simulink library "wheelSpeed_lib"  (R2023b)
settings: Solver=VariableStepAuto  StartTime=0.0  StopTime=10.0  RelTol=1e-3
undefined symbols (not defined in the file): raptor_xcp_function
libraries: Raptor_lib x50, simulink x6, $bdroot x4
settings Model: Creator=serga  LastModifiedBy=serga
settings OptimizationCC: ReuseModelBlockBuffer=off

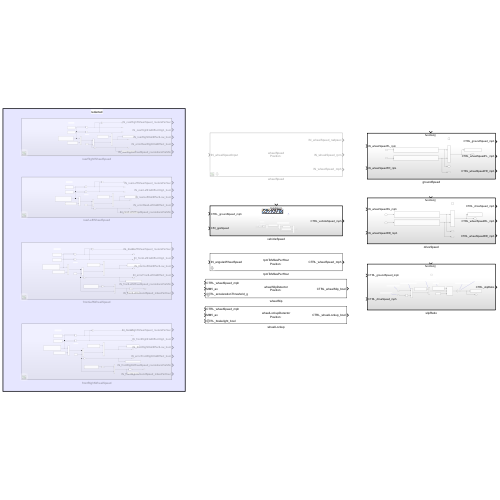
[thumbnail: Simulink's stored preview of the top-level diagram]
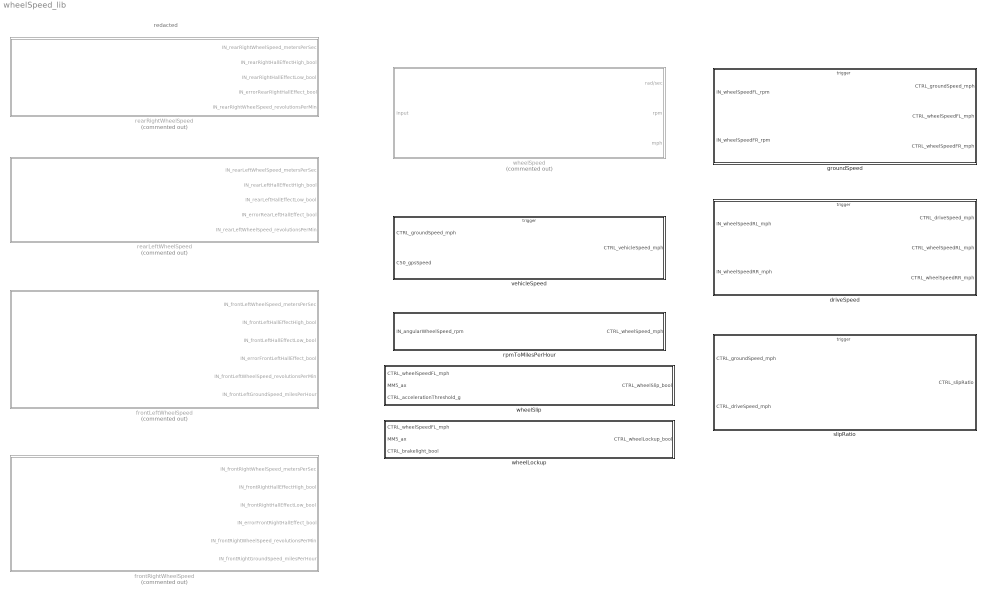
== system wheelSpeed_lib ==
  note: redacted
  driveSpeed : Subsystem  TreatAsAtomicUnit=on
  frontLeftWheelSpeed : Subsystem  Commented=on
  frontRightWheelSpeed : Subsystem  Commented=on
  groundSpeed : Subsystem  TreatAsAtomicUnit=on
  rearLeftWheelSpeed : Subsystem  Commented=on
  rearRightWheelSpeed : Subsystem  Commented=on
  rpmToMilesPerHour : Subsystem  mask{pos=''}
      mask prompts: pos "Position"
      mask Display:
      | disp(['rpmToMilesPerHour\n' ...
      |     'Position: ' pos]);
      | port_label('input', 1, ['IN_angularWheelSpeed' pos]);
      | port_label('output', 1, ['CTRL_wheelSpeed' pos '_mph']);
  slipRatio : Subsystem  TreatAsAtomicUnit=on
  vehicleSpeed : Subsystem
  wheelLockup : Subsystem  mask{pos=''}
      mask prompts: pos "Position"
      mask Display:
      | disp(['wheelLockupDetector\n' ...
      |     'Position: ' pos]);
      | port_label('input', 1, ['CTRL_wheelSpeed' pos '_mph']);
      | port_label('input', 2, 'MM5_ax');
      | port_label('input', 3, 'CTRL_brakelight_bool');
      | port_label('output', 1, ['CTRL_wheelLockup' pos '_bool']);
  wheelSlip : Subsystem  mask{pos=''}
      mask prompts: pos "Position"
      mask Display:
      | disp(['wheelSlipDetector\n' ...
      |     'Position: ' pos]);
      | port_label('input', 1, ['CTRL_wheelSpeed' pos '_mph']);
      | port_label('input', 2, 'MM5_ax');
      | port_label('input', 3, 'CTRL_accelerationThreshold_g');
      | port_label('output', 1, ['CTRL_wheelSlip' pos '_bool']);
  wheelSpeed : Subsystem  Commented=on  mask{pos=''}
      mask prompts: pos "Position"
      mask Display:
      | disp(['wheelSpeed\n' ...
      |     'Position: ' pos]);
      | port_label('input', 1, ['IN_wheelSpeedInput' pos]);
      | port_label('output', 1, ['IN_wheelSpeed' pos '_radpsec']);
      | port_label('output', 2, ['IN_wheelSpeed' pos '_rpm']);
      | port_label('output', 3, ['IN_wheelSpeed' pos '_mph']);

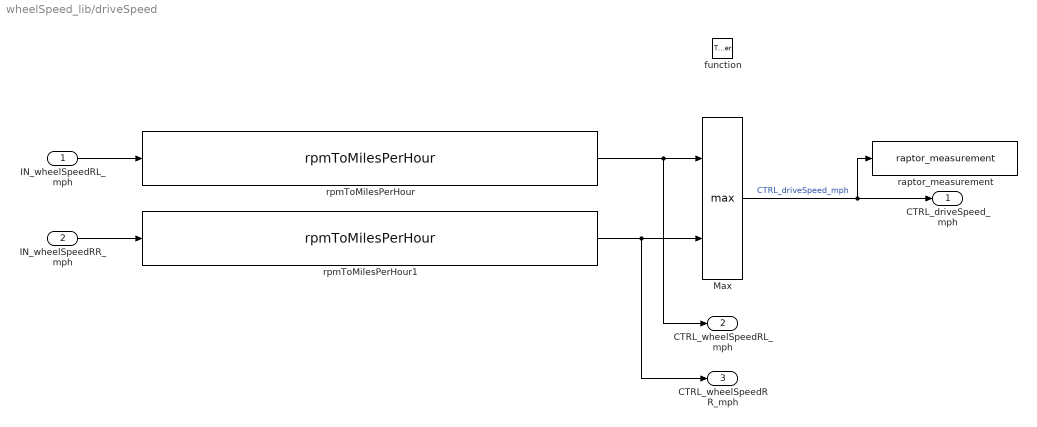
== system wheelSpeed_lib/driveSpeed ==
  IN_wheelSpeedRL_mph : Inport
  IN_wheelSpeedRR_mph : Inport  Port=2
  function : TriggerPort  TriggerType=function-call  VariantControl=(inherit)
  Max : MinMax  Function=max  Inputs=2
  raptor_measurement : Raptor_lib/Data Storage/raptor_measurement  paramName='DataName'  nameSource=Input Wire  calDispType=Number  calEnum={'False', 'True'}  calGain=1.0  calOffset=0.0  calMax=inf  calMin=-inf  calFormat='-1'  calUnit=''  calHelp=''  calAccess=1  calFunction=raptor_xcp_function(gcb)  calVisible=on
      settings: SourceProductName=Raptor
  rpmToMilesPerHour : $bdroot/rpmToMilesPerHour  pos='RL'
  rpmToMilesPerHour1 : $bdroot/rpmToMilesPerHour  pos='RR'
  CTRL_driveSpeed_mph : Outport
  CTRL_wheelSpeedRL_mph : Outport  Port=2
  CTRL_wheelSpeedRR_mph : Outport  Port=3
  wires:
  Max/1 -> raptor_measurement/1, CTRL_driveSpeed_mph/1  "CTRL_driveSpeed_mph"
  rpmToMilesPerHour/1 -> CTRL_wheelSpeedRL_mph/1, Max/1
  IN_wheelSpeedRL_mph/1 -> rpmToMilesPerHour/1
  rpmToMilesPerHour1/1 -> CTRL_wheelSpeedRR_mph/1, Max/2
  IN_wheelSpeedRR_mph/1 -> rpmToMilesPerHour1/1

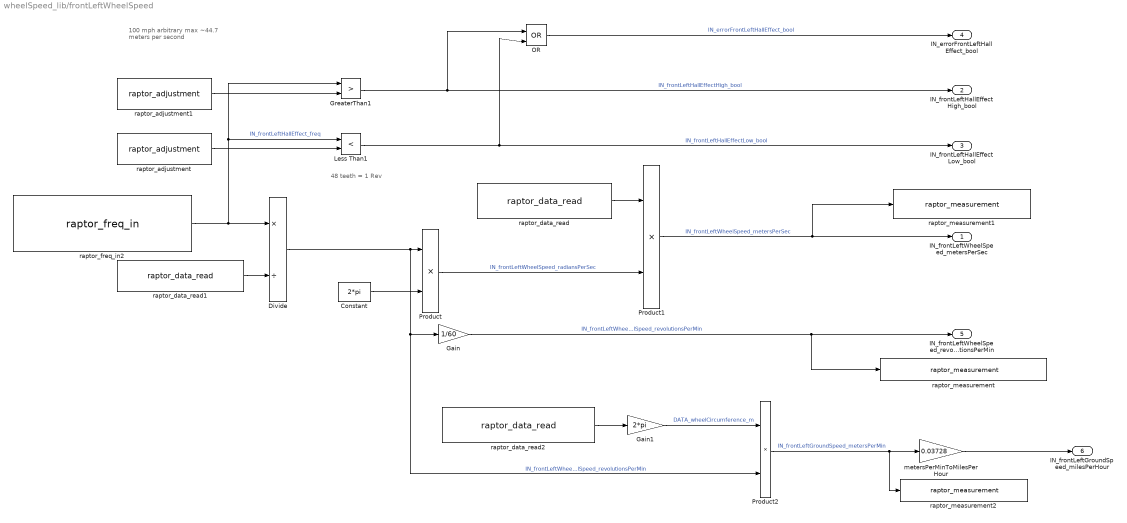
== system wheelSpeed_lib/frontLeftWheelSpeed ==
  note: 48 teeth = 1 Rev
  note: 100 mph arbitrary max
      | ~44.7 meters per second
  Constant : Constant  Value=2*pi
  Divide : Product  Inputs=*/
  Gain : Gain  Gain=1/60
  Gain1 : Gain  Gain=2*pi
  GreaterThan1 : RelationalOperator  Operator=>  OutDataTypeStr=boolean  RndMeth=Simplest  InputSameDT=off
  Less Than1 : RelationalOperator  Operator=<  OutDataTypeStr=boolean  RndMeth=Simplest  InputSameDT=off
  OR : Logic  Operator=OR  IconShape=distinctive  AllPortsSameDT=off  OutDataTypeStr=boolean
  Product : Product
  Product1 : Product
  Product2 : Product
  metersPerMinToMilesPerHour : Gain  Gain=0.03728
  raptor_adjustment : Raptor_lib/Data Storage/raptor_adjustment  paramName='IN_frontLeftHallEffectLow_freq'  nameSource=Parameter  initValue=0  dataType=single  storage=Calibration  calDispType=Number  calEnum={'False', 'True'}  calGain=1.0  calOffset=0.0  calMax=inf  calMin=-inf  calFormat='-1'  calUnit=''  calHelp=''  calAccess=1  calFunction=raptor_xcp_function(gcb)  calDispHeaders=off  calColHeaders={'Col1' 'Col2' 'Col3'}  calRowHeaders={'Row1' 'Row2' 'Row3'}
      settings: SourceProductName=Raptor
  raptor_adjustment1 : Raptor_lib/Data Storage/raptor_adjustment  paramName='IN_frontLeftHallEffectHigh_freq'  nameSource=Parameter  initValue=1680  dataType=single  storage=Calibration  calDispType=Number  calEnum={'False', 'True'}  calGain=1.0  calOffset=0.0  calMax=inf  calMin=-inf  calFormat='-1'  calUnit=''  calHelp=''  calAccess=1  calFunction=raptor_xcp_function(gcb)  calDispHeaders=off  calColHeaders={'Col1' 'Col2' 'Col3'}  calRowHeaders={'Row1' 'Row2' 'Row3'}
      settings: SourceProductName=Raptor
  raptor_data_read : Raptor_lib/Data Storage/raptor_data_read  dataName='DATA_unloadedWheelRadius_m'  dataShape=Scalar  idxSource=Input  idxRow=1  idxCol=1
      settings: SourceProductName=Raptor
  raptor_data_read1 : Raptor_lib/Data Storage/raptor_data_read  dataName='DATA_wheelTooth_ct'  dataShape=Scalar  idxSource=Input  idxRow=1  idxCol=1
      settings: SourceProductName=Raptor
  raptor_data_read2 : Raptor_lib/Data Storage/raptor_data_read  dataName='DATA_unloadedWheelRadius_m'  dataShape=Scalar  idxSource=Input  idxRow=1  idxCol=1
      settings: SourceProductName=Raptor
  raptor_freq_in2 : Raptor_lib/Input & Output/raptor_freq_in  minFreq='RAPTOR MASK DEFAULT'  resourceValues=INPUT41|INPUT42|INPUT43|INPUT44|INPUT45|(None)  resource=INPUT43  pullUDValues=[]  pullUD=[]  interfaceValues=[]  interface=[]  hasDuty=off  hasEdgeCount='RAPTOR MASK DEFAULT'
      settings: SourceProductName=Raptor
  raptor_measurement : Raptor_lib/Data Storage/raptor_measurement  paramName='DataName'  nameSource=Input Wire  calDispType=Number  calEnum={'False', 'True'}  calGain=1.0  calOffset=0.0  calMax=inf  calMin=-inf  calFormat='-1'  calUnit=''  calHelp=''  calAccess=1  calFunction=raptor_xcp_function(gcb)  calVisible=on
      settings: SourceProductName=Raptor
  raptor_measurement1 : Raptor_lib/Data Storage/raptor_measurement  paramName='DataName'  nameSource=Input Wire  calDispType=Number  calEnum={'False', 'True'}  calGain=1.0  calOffset=0.0  calMax=inf  calMin=-inf  calFormat='-1'  calUnit=''  calHelp=''  calAccess=1  calFunction=raptor_xcp_function(gcb)  calVisible=on
      settings: SourceProductName=Raptor
  raptor_measurement2 : Raptor_lib/Data Storage/raptor_measurement  paramName='DataName'  nameSource=Input Wire  calDispType=Number  calEnum={'False', 'True'}  calGain=1.0  calOffset=0.0  calMax=inf  calMin=-inf  calFormat='-1'  calUnit=''  calHelp=''  calAccess=1  calFunction=raptor_xcp_function(gcb)  calVisible=on
      settings: SourceProductName=Raptor
  IN_frontLeftWheelSpeed_metersPerSec : Outport
  IN_frontLeftHallEffectHigh_bool : Outport  Port=2
  IN_frontLeftHallEffectLow_bool : Outport  Port=3
  IN_errorFrontLeftHallEffect_bool : Outport  Port=4
  IN_frontLeftWheelSpeed_revolutionsPerMin : Outport  Port=5
  IN_frontLeftGroundSpeed_milesPerHour : Outport  Port=6
  wires:
  Product2/1 -> raptor_measurement2/1, metersPerMinToMilesPerHour/1  "IN_frontLeftGroundSpeed_metersPerMin"
  Divide/1 -> Product2/2, Gain/1, Product/1  "IN_frontLeftWheelSpeed_revolutionsPerMin"
  Gain1/1 -> Product2/1  "DATA_wheelCircumference_m"
  raptor_data_read/1 -> Product1/1
  raptor_data_read2/1 -> Gain1/1
  Less Than1/1 -> IN_frontLeftHallEffectLow_bool/1, OR/2  "IN_frontLeftHallEffectLow_bool"
  raptor_freq_in2/1 -> Less Than1/1, GreaterThan1/1, Divide/1  "IN_frontLeftHallEffect_freq"
  metersPerMinToMilesPerHour/1 -> IN_frontLeftGroundSpeed_milesPerHour/1
  Constant/1 -> Product/2
  raptor_adjustment/1 -> Less Than1/2
  OR/1 -> IN_errorFrontLeftHallEffect_bool/1  "IN_errorFrontLeftHallEffect_bool"
  raptor_adjustment1/1 -> GreaterThan1/2
  raptor_data_read1/1 -> Divide/2
  Product1/1 -> raptor_measurement1/1, IN_frontLeftWheelSpeed_metersPerSec/1  "IN_frontLeftWheelSpeed_metersPerSec"
  Gain/1 -> raptor_measurement/1, IN_frontLeftWheelSpeed_revolutionsPerMin/1  "IN_frontLeftWheelSpeed_revolutionsPerMin"
  Product/1 -> Product1/2  "IN_frontLeftWheelSpeed_radiansPerSec"
  GreaterThan1/1 -> IN_frontLeftHallEffectHigh_bool/1, OR/1  "IN_frontLeftHallEffectHigh_bool"

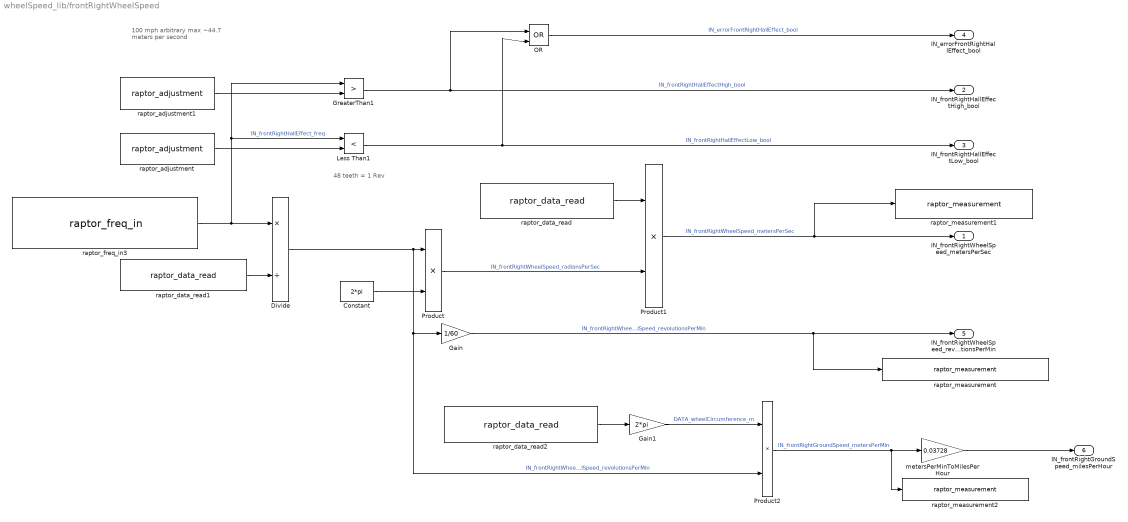
== system wheelSpeed_lib/frontRightWheelSpeed ==
  note: 100 mph arbitrary max
      | ~44.7 meters per second
  note: 48 teeth = 1 Rev
  Constant : Constant  Value=2*pi
  Divide : Product  Inputs=*/
  Gain : Gain  Gain=1/60
  Gain1 : Gain  Gain=2*pi
  GreaterThan1 : RelationalOperator  Operator=>  OutDataTypeStr=boolean  RndMeth=Simplest  InputSameDT=off
  Less Than1 : RelationalOperator  Operator=<  OutDataTypeStr=boolean  RndMeth=Simplest  InputSameDT=off
  OR : Logic  Operator=OR  IconShape=distinctive  AllPortsSameDT=off  OutDataTypeStr=boolean
  Product : Product
  Product1 : Product
  Product2 : Product
  metersPerMinToMilesPerHour : Gain  Gain=0.03728
  raptor_adjustment : Raptor_lib/Data Storage/raptor_adjustment  paramName='IN_frontRightHallEffectLow_freq'  nameSource=Parameter  initValue=0  dataType=single  storage=Calibration  calDispType=Number  calEnum={'False', 'True'}  calGain=1.0  calOffset=0.0  calMax=inf  calMin=-inf  calFormat='-1'  calUnit=''  calHelp=''  calAccess=1  calFunction=raptor_xcp_function(gcb)  calDispHeaders=off  calColHeaders={'Col1' 'Col2' 'Col3'}  calRowHeaders={'Row1' 'Row2' 'Row3'}
      settings: SourceProductName=Raptor
  raptor_adjustment1 : Raptor_lib/Data Storage/raptor_adjustment  paramName='IN_frontRightHallEffectHigh_freq'  nameSource=Parameter  initValue=1680  dataType=single  storage=Calibration  calDispType=Number  calEnum={'False', 'True'}  calGain=1.0  calOffset=0.0  calMax=inf  calMin=-inf  calFormat='-1'  calUnit=''  calHelp=''  calAccess=1  calFunction=raptor_xcp_function(gcb)  calDispHeaders=off  calColHeaders={'Col1' 'Col2' 'Col3'}  calRowHeaders={'Row1' 'Row2' 'Row3'}
      settings: SourceProductName=Raptor
  raptor_data_read : Raptor_lib/Data Storage/raptor_data_read  dataName='DATA_unloadedWheelRadius_m'  dataShape=Scalar  idxSource=Input  idxRow=1  idxCol=1
      settings: SourceProductName=Raptor
  raptor_data_read1 : Raptor_lib/Data Storage/raptor_data_read  dataName='DATA_wheelTooth_ct'  dataShape=Scalar  idxSource=Input  idxRow=1  idxCol=1
      settings: SourceProductName=Raptor
  raptor_data_read2 : Raptor_lib/Data Storage/raptor_data_read  dataName='DATA_unloadedWheelRadius_m'  dataShape=Scalar  idxSource=Input  idxRow=1  idxCol=1
      settings: SourceProductName=Raptor
  raptor_freq_in3 : Raptor_lib/Input & Output/raptor_freq_in  minFreq='RAPTOR MASK DEFAULT'  resourceValues=INPUT41|INPUT42|INPUT43|INPUT44|INPUT45|(None)  resource=INPUT44  pullUDValues=[]  pullUD=[]  interfaceValues=[]  interface=[]  hasDuty=off  hasEdgeCount='RAPTOR MASK DEFAULT'
      settings: SourceProductName=Raptor
  raptor_measurement : Raptor_lib/Data Storage/raptor_measurement  paramName='DataName'  nameSource=Input Wire  calDispType=Number  calEnum={'False', 'True'}  calGain=1.0  calOffset=0.0  calMax=inf  calMin=-inf  calFormat='-1'  calUnit=''  calHelp=''  calAccess=1  calFunction=raptor_xcp_function(gcb)  calVisible=on
      settings: SourceProductName=Raptor
  raptor_measurement1 : Raptor_lib/Data Storage/raptor_measurement  paramName='DataName'  nameSource=Input Wire  calDispType=Number  calEnum={'False', 'True'}  calGain=1.0  calOffset=0.0  calMax=inf  calMin=-inf  calFormat='-1'  calUnit=''  calHelp=''  calAccess=1  calFunction=raptor_xcp_function(gcb)  calVisible=on
      settings: SourceProductName=Raptor
  raptor_measurement2 : Raptor_lib/Data Storage/raptor_measurement  paramName='DataName'  nameSource=Input Wire  calDispType=Number  calEnum={'False', 'True'}  calGain=1.0  calOffset=0.0  calMax=inf  calMin=-inf  calFormat='-1'  calUnit=''  calHelp=''  calAccess=1  calFunction=raptor_xcp_function(gcb)  calVisible=on
      settings: SourceProductName=Raptor
  IN_frontRightWheelSpeed_metersPerSec : Outport
  IN_frontRightHallEffectHigh_bool : Outport  Port=2
  IN_frontRightHallEffectLow_bool : Outport  Port=3
  IN_errorFrontRightHallEffect_bool : Outport  Port=4
  IN_frontRightWheelSpeed_revolutionsPerMin : Outport  Port=5
  IN_frontRightGroundSpeed_milesPerHour : Outport  Port=6
  wires:
  raptor_adjustment/1 -> Less Than1/2
  raptor_freq_in3/1 -> Less Than1/1, GreaterThan1/1, Divide/1  "IN_frontRightHallEffect_freq"
  raptor_adjustment1/1 -> GreaterThan1/2
  OR/1 -> IN_errorFrontRightHallEffect_bool/1  "IN_errorFrontRightHallEffect_bool"
  GreaterThan1/1 -> IN_frontRightHallEffectHigh_bool/1, OR/1  "IN_frontRightHallEffectHigh_bool"
  Less Than1/1 -> IN_frontRightHallEffectLow_bool/1, OR/2  "IN_frontRightHallEffectLow_bool"
  Gain/1 -> raptor_measurement/1, IN_frontRightWheelSpeed_revolutionsPerMin/1  "IN_frontRightWheelSpeed_revolutionsPerMin"
  raptor_data_read1/1 -> Divide/2
  raptor_data_read/1 -> Product1/1
  Constant/1 -> Product/2
  Product1/1 -> raptor_measurement1/1, IN_frontRightWheelSpeed_metersPerSec/1  "IN_frontRightWheelSpeed_metersPerSec"
  Product/1 -> Product1/2  "IN_frontRightWheelSpeed_radiansPerSec"
  Product2/1 -> raptor_measurement2/1, metersPerMinToMilesPerHour/1  "IN_frontRightGroundSpeed_metersPerMin"
  Gain1/1 -> Product2/1  "DATA_wheelCircumference_m"
  Divide/1 -> Product2/2, Gain/1, Product/1  "IN_frontRightWheelSpeed_revolutionsPerMin"
  raptor_data_read2/1 -> Gain1/1
  metersPerMinToMilesPerHour/1 -> IN_frontRightGroundSpeed_milesPerHour/1

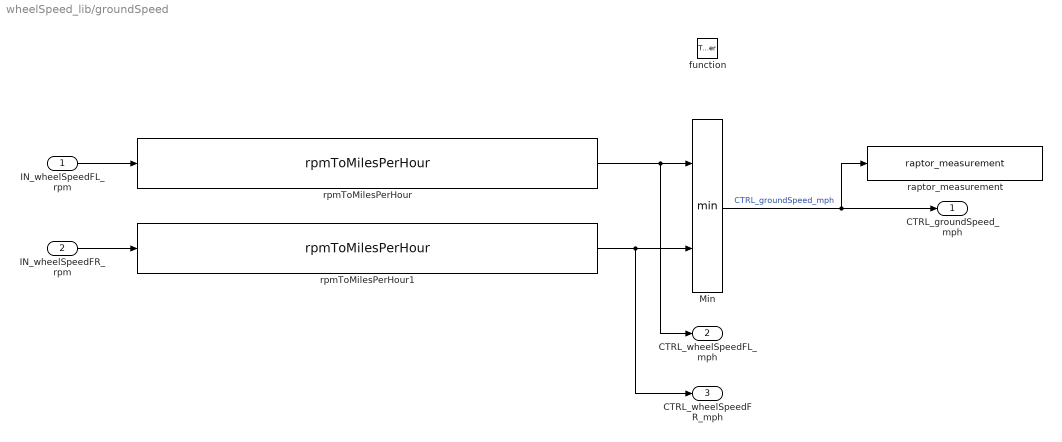
== system wheelSpeed_lib/groundSpeed ==
  IN_wheelSpeedFL_rpm : Inport
  IN_wheelSpeedFR_rpm : Inport  Port=2
  function : TriggerPort  TriggerType=function-call  VariantControl=(inherit)
  Min : MinMax  Inputs=2
  raptor_measurement : Raptor_lib/Data Storage/raptor_measurement  paramName='DataName'  nameSource=Input Wire  calDispType=Number  calEnum={'False', 'True'}  calGain=1.0  calOffset=0.0  calMax=inf  calMin=-inf  calFormat='-1'  calUnit=''  calHelp=''  calAccess=1  calFunction=raptor_xcp_function(gcb)  calVisible=on
      settings: SourceProductName=Raptor
  rpmToMilesPerHour : $bdroot/rpmToMilesPerHour  pos='FL'
  rpmToMilesPerHour1 : $bdroot/rpmToMilesPerHour  pos='FR'
  CTRL_groundSpeed_mph : Outport
  CTRL_wheelSpeedFL_mph : Outport  Port=2
  CTRL_wheelSpeedFR_mph : Outport  Port=3
  wires:
  Min/1 -> raptor_measurement/1, CTRL_groundSpeed_mph/1  "CTRL_groundSpeed_mph"
  rpmToMilesPerHour/1 -> CTRL_wheelSpeedFL_mph/1, Min/1
  rpmToMilesPerHour1/1 -> CTRL_wheelSpeedFR_mph/1, Min/2
  IN_wheelSpeedFL_rpm/1 -> rpmToMilesPerHour/1
  IN_wheelSpeedFR_rpm/1 -> rpmToMilesPerHour1/1

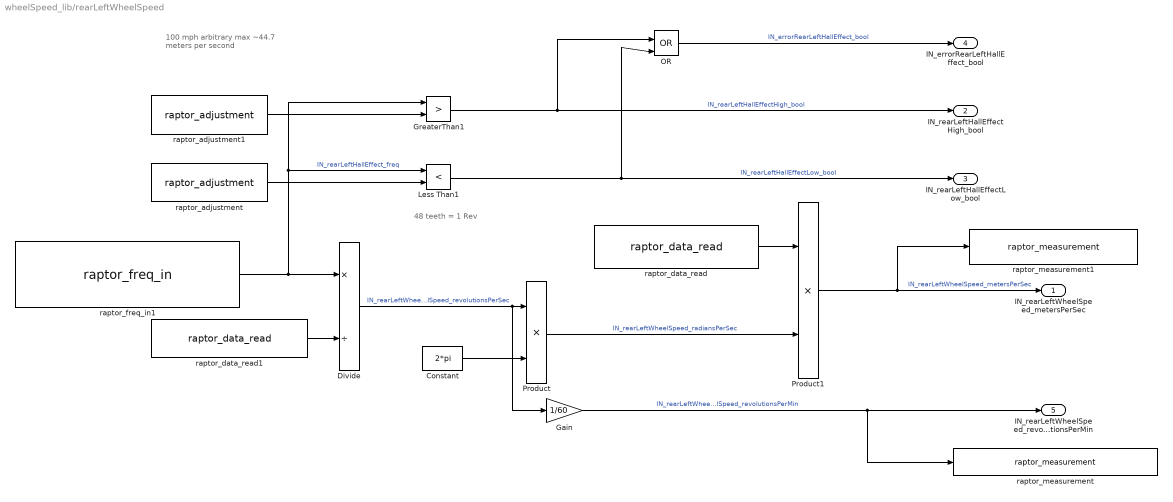
== system wheelSpeed_lib/rearLeftWheelSpeed ==
  note: 100 mph arbitrary max
      | ~44.7 meters per second
  note: 48 teeth = 1 Rev
  Constant : Constant  Value=2*pi
  Divide : Product  Inputs=*/
  Gain : Gain  Gain=1/60
  GreaterThan1 : RelationalOperator  Operator=>  OutDataTypeStr=boolean  RndMeth=Simplest  InputSameDT=off
  Less Than1 : RelationalOperator  Operator=<  OutDataTypeStr=boolean  RndMeth=Simplest  InputSameDT=off
  OR : Logic  Operator=OR  IconShape=distinctive  AllPortsSameDT=off  OutDataTypeStr=boolean
  Product : Product
  Product1 : Product
  raptor_adjustment : Raptor_lib/Data Storage/raptor_adjustment  paramName='IN_rearLeftHallEffectLow_freq'  nameSource=Parameter  initValue=0  dataType=single  storage=Calibration  calDispType=Number  calEnum={'False', 'True'}  calGain=1.0  calOffset=0.0  calMax=inf  calMin=-inf  calFormat='-1'  calUnit=''  calHelp=''  calAccess=1  calFunction=raptor_xcp_function(gcb)  calDispHeaders=off  calColHeaders={'Col1' 'Col2' 'Col3'}  calRowHeaders={'Row1' 'Row2' 'Row3'}
      settings: SourceProductName=Raptor
  raptor_adjustment1 : Raptor_lib/Data Storage/raptor_adjustment  paramName='IN_rearLeftHallEffectHigh_freq'  nameSource=Parameter  initValue=1680  dataType=single  storage=Calibration  calDispType=Number  calEnum={'False', 'True'}  calGain=1.0  calOffset=0.0  calMax=inf  calMin=-inf  calFormat='-1'  calUnit=''  calHelp=''  calAccess=1  calFunction=raptor_xcp_function(gcb)  calDispHeaders=off  calColHeaders={'Col1' 'Col2' 'Col3'}  calRowHeaders={'Row1' 'Row2' 'Row3'}
      settings: SourceProductName=Raptor
  raptor_data_read : Raptor_lib/Data Storage/raptor_data_read  dataName='DATA_unloadedWheelRadius_m'  dataShape=Scalar  idxSource=Input  idxRow=1  idxCol=1
      settings: SourceProductName=Raptor
  raptor_data_read1 : Raptor_lib/Data Storage/raptor_data_read  dataName='DATA_wheelTooth_ct'  dataShape=Scalar  idxSource=Input  idxRow=1  idxCol=1
      settings: SourceProductName=Raptor
  raptor_freq_in1 : Raptor_lib/Input & Output/raptor_freq_in  minFreq='RAPTOR MASK DEFAULT'  resourceValues=INPUT41|INPUT42|INPUT43|INPUT44|INPUT45|(None)  resource=INPUT42  pullUDValues=[]  pullUD=[]  interfaceValues=[]  interface=[]  hasDuty=off  hasEdgeCount='RAPTOR MASK DEFAULT'
      settings: SourceProductName=Raptor
  raptor_measurement : Raptor_lib/Data Storage/raptor_measurement  paramName='DataName'  nameSource=Input Wire  calDispType=Number  calEnum={'False', 'True'}  calGain=1.0  calOffset=0.0  calMax=inf  calMin=-inf  calFormat='-1'  calUnit=''  calHelp=''  calAccess=1  calFunction=raptor_xcp_function(gcb)  calVisible=on
      settings: SourceProductName=Raptor
  raptor_measurement1 : Raptor_lib/Data Storage/raptor_measurement  paramName='DataName'  nameSource=Input Wire  calDispType=Number  calEnum={'False', 'True'}  calGain=1.0  calOffset=0.0  calMax=inf  calMin=-inf  calFormat='-1'  calUnit=''  calHelp=''  calAccess=1  calFunction=raptor_xcp_function(gcb)  calVisible=on
      settings: SourceProductName=Raptor
  IN_rearLeftWheelSpeed_metersPerSec : Outport
  IN_rearLeftHallEffectHigh_bool : Outport  Port=2
  IN_rearLeftHallEffectLow_bool : Outport  Port=3
  IN_errorRearLeftHallEffect_bool : Outport  Port=4
  IN_rearLeftWheelSpeed_revolutionsPerMin : Outport  Port=5
  wires:
  raptor_adjustment/1 -> Less Than1/2
  raptor_freq_in1/1 -> Less Than1/1, GreaterThan1/1, Divide/1  "IN_rearLeftHallEffect_freq"
  raptor_adjustment1/1 -> GreaterThan1/2
  OR/1 -> IN_errorRearLeftHallEffect_bool/1  "IN_errorRearLeftHallEffect_bool"
  GreaterThan1/1 -> IN_rearLeftHallEffectHigh_bool/1, OR/1  "IN_rearLeftHallEffectHigh_bool"
  Less Than1/1 -> IN_rearLeftHallEffectLow_bool/1, OR/2  "IN_rearLeftHallEffectLow_bool"
  Gain/1 -> IN_rearLeftWheelSpeed_revolutionsPerMin/1, raptor_measurement/1  "IN_rearLeftWheelSpeed_revolutionsPerMin"
  raptor_data_read1/1 -> Divide/2
  raptor_data_read/1 -> Product1/1
  Divide/1 -> Gain/1, Product/1  "IN_rearLeftWheelSpeed_revolutionsPerSec"
  Constant/1 -> Product/2
  Product1/1 -> raptor_measurement1/1, IN_rearLeftWheelSpeed_metersPerSec/1  "IN_rearLeftWheelSpeed_metersPerSec"
  Product/1 -> Product1/2  "IN_rearLeftWheelSpeed_radiansPerSec"

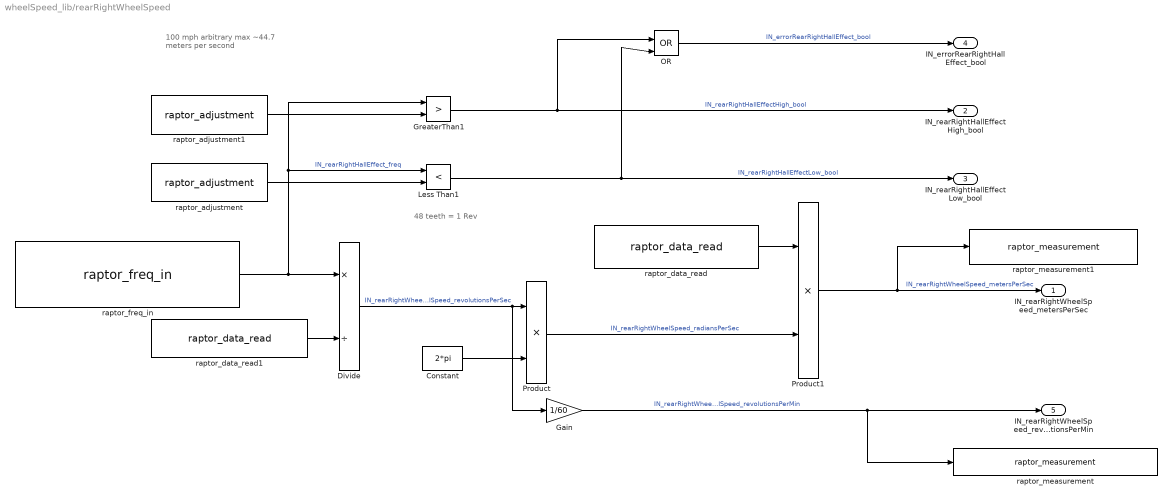
== system wheelSpeed_lib/rearRightWheelSpeed ==
  note: 100 mph arbitrary max
      | ~44.7 meters per second
  note: 48 teeth = 1 Rev
  Constant : Constant  Value=2*pi
  Divide : Product  Inputs=*/
  Gain : Gain  Gain=1/60
  GreaterThan1 : RelationalOperator  Operator=>  OutDataTypeStr=boolean  RndMeth=Simplest  InputSameDT=off
  Less Than1 : RelationalOperator  Operator=<  OutDataTypeStr=boolean  RndMeth=Simplest  InputSameDT=off
  OR : Logic  Operator=OR  IconShape=distinctive  AllPortsSameDT=off  OutDataTypeStr=boolean
  Product : Product
  Product1 : Product
  raptor_adjustment : Raptor_lib/Data Storage/raptor_adjustment  paramName='IN_rearRightHallEffectLow_freq'  nameSource=Parameter  initValue=0  dataType=single  storage=Calibration  calDispType=Number  calEnum={'False', 'True'}  calGain=1.0  calOffset=0.0  calMax=inf  calMin=-inf  calFormat='-1'  calUnit=''  calHelp=''  calAccess=1  calFunction=raptor_xcp_function(gcb)  calDispHeaders=off  calColHeaders={'Col1' 'Col2' 'Col3'}  calRowHeaders={'Row1' 'Row2' 'Row3'}
      settings: SourceProductName=Raptor
  raptor_adjustment1 : Raptor_lib/Data Storage/raptor_adjustment  paramName='IN_rearRightHallEffectHigh_freq'  nameSource=Parameter  initValue=1680  dataType=single  storage=Calibration  calDispType=Number  calEnum={'False', 'True'}  calGain=1.0  calOffset=0.0  calMax=inf  calMin=-inf  calFormat='-1'  calUnit=''  calHelp=''  calAccess=1  calFunction=raptor_xcp_function(gcb)  calDispHeaders=off  calColHeaders={'Col1' 'Col2' 'Col3'}  calRowHeaders={'Row1' 'Row2' 'Row3'}
      settings: SourceProductName=Raptor
  raptor_data_read : Raptor_lib/Data Storage/raptor_data_read  dataName='DATA_unloadedWheelRadius_m'  dataShape=Scalar  idxSource=Input  idxRow=1  idxCol=1
      settings: SourceProductName=Raptor
  raptor_data_read1 : Raptor_lib/Data Storage/raptor_data_read  dataName='DATA_wheelTooth_ct'  dataShape=Scalar  idxSource=Input  idxRow=1  idxCol=1
      settings: SourceProductName=Raptor
  raptor_freq_in : Raptor_lib/Input & Output/raptor_freq_in  minFreq='RAPTOR MASK DEFAULT'  resourceValues=INPUT41|INPUT42|INPUT43|INPUT44|INPUT45|(None)  resource=INPUT41  pullUDValues=[]  pullUD=[]  interfaceValues=[]  interface=[]  hasDuty=off  hasEdgeCount='RAPTOR MASK DEFAULT'
      settings: SourceProductName=Raptor
  raptor_measurement : Raptor_lib/Data Storage/raptor_measurement  paramName='DataName'  nameSource=Input Wire  calDispType=Number  calEnum={'False', 'True'}  calGain=1.0  calOffset=0.0  calMax=inf  calMin=-inf  calFormat='-1'  calUnit=''  calHelp=''  calAccess=1  calFunction=raptor_xcp_function(gcb)  calVisible=on
      settings: SourceProductName=Raptor
  raptor_measurement1 : Raptor_lib/Data Storage/raptor_measurement  paramName='DataName'  nameSource=Input Wire  calDispType=Number  calEnum={'False', 'True'}  calGain=1.0  calOffset=0.0  calMax=inf  calMin=-inf  calFormat='-1'  calUnit=''  calHelp=''  calAccess=1  calFunction=raptor_xcp_function(gcb)  calVisible=on
      settings: SourceProductName=Raptor
  IN_rearRightWheelSpeed_metersPerSec : Outport
  IN_rearRightHallEffectHigh_bool : Outport  Port=2
  IN_rearRightHallEffectLow_bool : Outport  Port=3
  IN_errorRearRightHallEffect_bool : Outport  Port=4
  IN_rearRightWheelSpeed_revolutionsPerMin : Outport  Port=5
  wires:
  raptor_data_read1/1 -> Divide/2
  Divide/1 -> Gain/1, Product/1  "IN_rearRightWheelSpeed_revolutionsPerSec"
  Constant/1 -> Product/2
  Product/1 -> Product1/2  "IN_rearRightWheelSpeed_radiansPerSec"
  raptor_data_read/1 -> Product1/1
  Product1/1 -> raptor_measurement1/1, IN_rearRightWheelSpeed_metersPerSec/1  "IN_rearRightWheelSpeed_metersPerSec"
  raptor_freq_in/1 -> Less Than1/1, GreaterThan1/1, Divide/1  "IN_rearRightHallEffect_freq"
  raptor_adjustment1/1 -> GreaterThan1/2
  raptor_adjustment/1 -> Less Than1/2
  Less Than1/1 -> IN_rearRightHallEffectLow_bool/1, OR/2  "IN_rearRightHallEffectLow_bool"
  OR/1 -> IN_errorRearRightHallEffect_bool/1  "IN_errorRearRightHallEffect_bool"
  GreaterThan1/1 -> IN_rearRightHallEffectHigh_bool/1, OR/1  "IN_rearRightHallEffectHigh_bool"
  Gain/1 -> IN_rearRightWheelSpeed_revolutionsPerMin/1, raptor_measurement/1  "IN_rearRightWheelSpeed_revolutionsPerMin"

== system wheelSpeed_lib/rpmToMilesPerHour ==
  note: meters to miles
  IN_angularWheelSpeed_rpm : Inport
  Gain : Gain  Gain=0.000621371
  Gain1 : Gain  Gain=60
  Product : Product
  raptor_data_read : Raptor_lib/Data Storage/raptor_data_read  dataName='DATA_unloadedWheelRadius_m'  dataShape=Scalar  idxSource=Input  idxRow=1  idxCol=1
      settings: SourceProductName=Raptor
  CTRL_wheelSpeed_mph : Outport
  wires:
  raptor_data_read/1 -> Gain/1
  IN_angularWheelSpeed_rpm/1 -> Product/2
  Gain/1 -> Product/1
  Product/1 -> Gain1/1
  Gain1/1 -> CTRL_wheelSpeed_mph/1

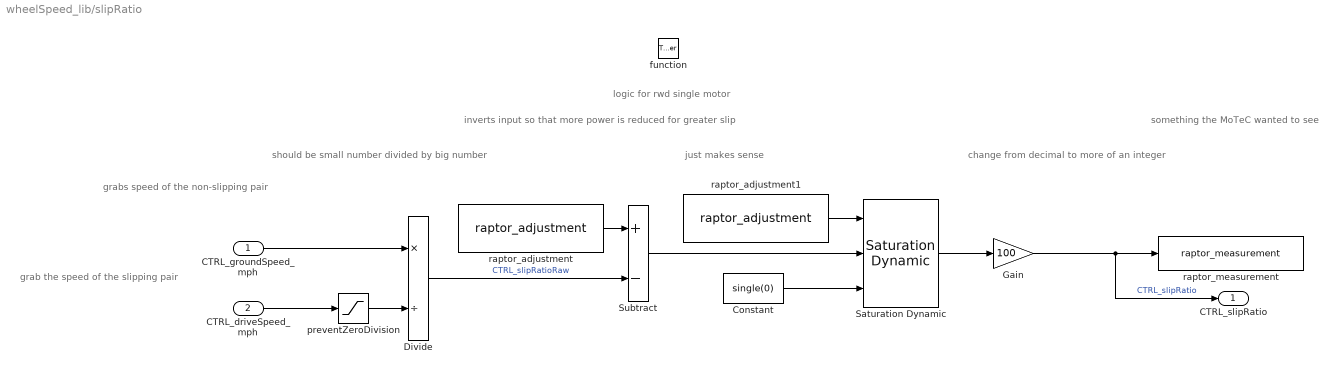
== system wheelSpeed_lib/slipRatio ==
  note: something the MoTeC wanted to see
  note: change from decimal to more of an integer
  note: inverts input so that more power is reduced for greater slip
  note: just makes sense
  note: logic for rwd single motor
  note: should be small number divided by big number
  note: grab the speed of the slipping pair
  note: grabs speed of the non-slipping pair
  CTRL_groundSpeed_mph : Inport
  CTRL_driveSpeed_mph : Inport  Port=2
  function : TriggerPort  TriggerType=function-call  VariantControl=(inherit)
  Constant : Constant  Value=single(0)
  Divide : Product  Inputs=*/
  Gain : Gain  Gain=100
  Saturation Dynamic : simulink/Discontinuities/Saturation Dynamic  OutMin=[]  OutMax=[]  OutDataTypeStr=Inherit: Same as second input  OutDataType=fixdt(1, 16)  OutScaling=2^-10  DoSatur=off
  Subtract : Sum  Inputs=+-
  preventZeroDivision : Saturate  UpperLimit=inf  LowerLimit=0.0001
      settings: AttributesFormatString=|
      | LL: %<LowerLimit>
      | UL: %<UpperLimit>
  raptor_adjustment : Raptor_lib/Data Storage/raptor_adjustment  paramName='CTRL_slipConstant'  nameSource=Parameter  initValue=1  dataType=double  storage=Calibration  calDispType=Number  calEnum={'False', 'True'}  calGain=1.0  calOffset=0.0  calMax=inf  calMin=-inf  calFormat='-1'  calUnit=''  calHelp=''  calAccess=1  calFunction=raptor_xcp_function(gcb)  calDispHeaders=off  calColHeaders={'Col1' 'Col2' 'Col3'}  calRowHeaders={'Row1' 'Row2' 'Row3'}
      settings: SourceProductName=Raptor
  raptor_adjustment1 : Raptor_lib/Data Storage/raptor_adjustment  paramName='CTRL_slipRatioUpperThresh'  nameSource=Parameter  initValue=1  dataType=single  storage=Calibration  calDispType=Number  calEnum={'False', 'True'}  calGain=1.0  calOffset=0.0  calMax=inf  calMin=-inf  calFormat='-1'  calUnit=''  calHelp=''  calAccess=1  calFunction=raptor_xcp_function(gcb)  calDispHeaders=off  calColHeaders={'Col1' 'Col2' 'Col3'}  calRowHeaders={'Row1' 'Row2' 'Row3'}
      settings: SourceProductName=Raptor
  raptor_measurement : Raptor_lib/Data Storage/raptor_measurement  paramName='DataName'  nameSource=Input Wire  calDispType=Number  calEnum={'False', 'True'}  calGain=1.0  calOffset=0.0  calMax=inf  calMin=-inf  calFormat='-1'  calUnit=''  calHelp=''  calAccess=1  calFunction=raptor_xcp_function(gcb)  calVisible=on
      settings: SourceProductName=Raptor
  CTRL_slipRatio : Outport
  wires:
  CTRL_groundSpeed_mph/1 -> Divide/1
  CTRL_driveSpeed_mph/1 -> preventZeroDivision/1
  preventZeroDivision/1 -> Divide/2
  Divide/1 -> Subtract/2  "CTRL_slipRatioRaw"
  raptor_adjustment/1 -> Subtract/1
  Subtract/1 -> Saturation Dynamic/2
  Saturation Dynamic/1 -> Gain/1
  raptor_adjustment1/1 -> Saturation Dynamic/1
  Constant/1 -> Saturation Dynamic/3
  Gain/1 -> CTRL_slipRatio/1, raptor_measurement/1  "CTRL_slipRatio"

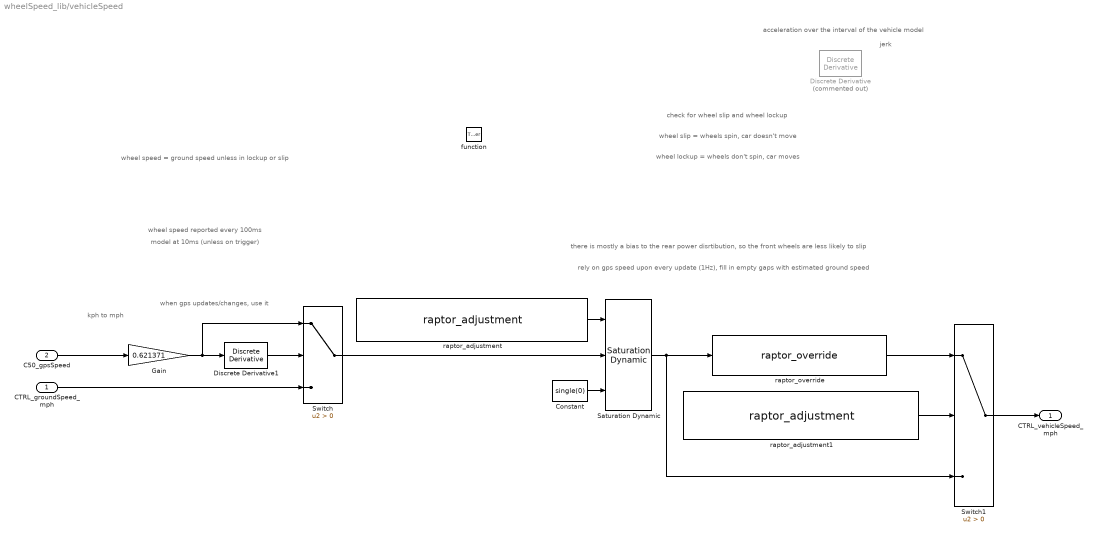
== system wheelSpeed_lib/vehicleSpeed ==
  note: model at 10ms (unless on trigger)
  note: wheel speed reported every 100ms
  note: jerk
  note: wheel speed = ground speed unless in lockup or slip
  note: acceleration over the interval of the vehicle model
  note: wheel slip = wheels spin, car doesn't move
  note: when gps updates/changes, use it
  note: rely on gps speed upon every update (1Hz), fill in empty gaps with estimated ground speed
  note: wheel lockup = wheels don't spin, car moves
  note: kph to mph
  note: there is mostly a bias to the rear power disrtibution, so the front wheels are less likely to slip
  note: check for wheel slip and wheel lockup
  CTRL_groundSpeed_mph : Inport
  C50_gpsSpeed : Inport  Port=2
  function : TriggerPort  TriggerType=function-call  VariantControl=(inherit)
  Constant : Constant  Value=single(0)
  Discrete Derivative : simulink/Discrete/Discrete Derivative  Commented=on  gainval=1.0  ICPrevScaledInput=0.0  OutMin=[]  OutMax=[]  OutDataType=fixdt(1, 16)  OutScaling=2^-10  DoSatur=off
  Discrete Derivative1 : simulink/Discrete/Discrete Derivative  gainval=1.0  ICPrevScaledInput=0.0  OutMin=[]  OutMax=[]  OutDataType=fixdt(1, 16)  OutScaling=2^-10  DoSatur=off
  Gain : Gain  Gain=0.621371
  Saturation Dynamic : simulink/Discontinuities/Saturation Dynamic  OutMin=[]  OutMax=[]  OutDataTypeStr=Inherit: Same as second input  OutDataType=fixdt(1, 16)  OutScaling=2^-10  DoSatur=off
  Switch : Switch  Criteria=u2 > Threshold  SaturateOnIntegerOverflow=off  InputSameDT=off
  Switch1 : Switch  Criteria=u2 > Threshold  SaturateOnIntegerOverflow=off  InputSameDT=off
  raptor_adjustment : Raptor_lib/Data Storage/raptor_adjustment  paramName='CTRL_vehicleSpeedUpperThresh_mph'  nameSource=Parameter  initValue=100  dataType=single  storage=Calibration  calDispType=Number  calEnum={'False', 'True'}  calGain=1.0  calOffset=0.0  calMax=inf  calMin=-inf  calFormat='-1'  calUnit=''  calHelp=''  calAccess=1  calFunction=raptor_xcp_function(gcb)  calDispHeaders=off  calColHeaders={'Col1' 'Col2' 'Col3'}  calRowHeaders={'Row1' 'Row2' 'Row3'}
      settings: SourceProductName=Raptor
  raptor_adjustment1 : Raptor_lib/Data Storage/raptor_adjustment  paramName='CTRL_vehicleSpeedOverride_bool'  nameSource=Parameter  initValue=0  dataType=boolean  storage=Calibration  calDispType=Number  calEnum={'False', 'True'}  calGain=1.0  calOffset=0.0  calMax=inf  calMin=-inf  calFormat='-1'  calUnit=''  calHelp=''  calAccess=1  calFunction=raptor_xcp_function(gcb)  calDispHeaders=off  calColHeaders={'Col1' 'Col2' 'Col3'}  calRowHeaders={'Row1' 'Row2' 'Row3'}
      settings: SourceProductName=Raptor
  raptor_override : Raptor_lib/Data Storage/raptor_override  paramName='CTRL_vehicleSpeedOverride_mph'  nameSource=Parameter  measurement=None  calDispType=Number  calEnum={'False', 'True'}  calGain=1.0  calOffset=0.0  calMax=inf  calMin=-inf  calFormat='-1'  calUnit=''  calHelp=''  calAccess=1  calFunction="[raptor_xcp_function(gcb) '|'  'Override']"
      settings: SourceProductName=Raptor
  CTRL_vehicleSpeed_mph : Outport
  wires:
  Saturation Dynamic/1 -> Switch1/3, raptor_override/1
  Switch/1 -> Saturation Dynamic/2
  raptor_adjustment1/1 -> Switch1/2
  raptor_override/1 -> Switch1/1
  Switch1/1 -> CTRL_vehicleSpeed_mph/1
  raptor_adjustment/1 -> Saturation Dynamic/1
  Gain/1 -> Switch/1, Discrete Derivative1/1
  Constant/1 -> Saturation Dynamic/3
  Discrete Derivative1/1 -> Switch/2
  CTRL_groundSpeed_mph/1 -> Switch/3
  C50_gpsSpeed/1 -> Gain/1

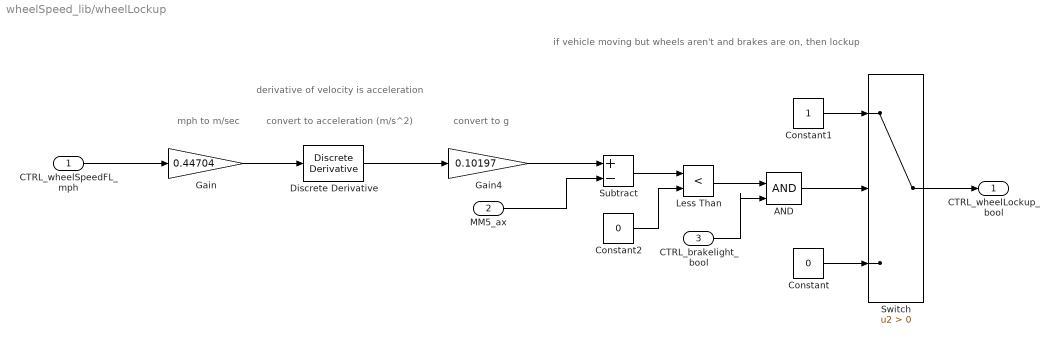
== system wheelSpeed_lib/wheelLockup ==
  note: mph to m/sec
  note: convert to g
  note: convert to acceleration (m/s^2)
  note: derivative of velocity is acceleration
  note: if vehicle moving but wheels aren't and brakes are on, then lockup
  CTRL_wheelSpeedFL_mph : Inport
  MM5_ax : Inport  Port=2
  CTRL_brakelight_bool : Inport  Port=3
  AND : Logic  IconShape=distinctive  AllPortsSameDT=off  OutDataTypeStr=boolean
  Constant : Constant  Value=0
  Constant1 : Constant
  Constant2 : Constant  Value=0
  Discrete Derivative : simulink/Discrete/Discrete Derivative  gainval=1.0  ICPrevScaledInput=0.0  OutMin=[]  OutMax=[]  OutDataType=fixdt(1, 16)  OutScaling=2^-10  DoSatur=off
  Gain : Gain  Gain=0.44704
  Gain4 : Gain  Gain=0.10197
  Less Than : RelationalOperator  Operator=<  OutDataTypeStr=boolean  RndMeth=Simplest  InputSameDT=off
  Subtract : Sum  Inputs=+-
  Switch : Switch  Criteria=u2 > Threshold  SaturateOnIntegerOverflow=off  InputSameDT=off
  CTRL_wheelLockup_bool : Outport
  wires:
  Constant/1 -> Switch/3
  Switch/1 -> CTRL_wheelLockup_bool/1
  Discrete Derivative/1 -> Gain4/1
  Constant1/1 -> Switch/1
  CTRL_wheelSpeedFL_mph/1 -> Gain/1
  Subtract/1 -> Less Than/1
  Gain/1 -> Discrete Derivative/1
  Gain4/1 -> Subtract/1
  MM5_ax/1 -> Subtract/2
  Constant2/1 -> Less Than/2
  Less Than/1 -> AND/1
  CTRL_brakelight_bool/1 -> AND/2
  AND/1 -> Switch/2

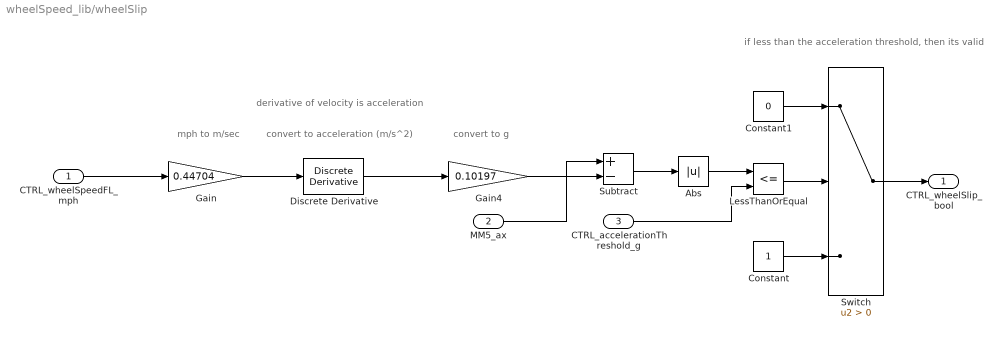
== system wheelSpeed_lib/wheelSlip ==
  note: if less than the acceleration threshold, then its valid
  note: convert to g
  note: convert to acceleration (m/s^2)
  note: mph to m/sec
  note: derivative of velocity is acceleration
  CTRL_wheelSpeedFL_mph : Inport
  MM5_ax : Inport  Port=2
  CTRL_accelerationThreshold_g : Inport  Port=3
  Abs : Abs  SaturateOnIntegerOverflow=off
  Constant : Constant
  Constant1 : Constant  Value=0
  Discrete Derivative : simulink/Discrete/Discrete Derivative  gainval=1.0  ICPrevScaledInput=0.0  OutMin=[]  OutMax=[]  OutDataType=fixdt(1, 16)  OutScaling=2^-10  DoSatur=off
  Gain : Gain  Gain=0.44704
  Gain4 : Gain  Gain=0.10197
  LessThanOrEqual : RelationalOperator  Operator=<=  OutDataTypeStr=boolean  RndMeth=Simplest  InputSameDT=off
  Subtract : Sum  Inputs=+-
  Switch : Switch  Criteria=u2 > Threshold  SaturateOnIntegerOverflow=off  InputSameDT=off
  CTRL_wheelSlip_bool : Outport
  wires:
  CTRL_wheelSpeedFL_mph/1 -> Gain/1
  MM5_ax/1 -> Subtract/1
  Discrete Derivative/1 -> Gain4/1
  Gain/1 -> Discrete Derivative/1
  Gain4/1 -> Subtract/2
  Subtract/1 -> Abs/1
  Abs/1 -> LessThanOrEqual/1
  CTRL_accelerationThreshold_g/1 -> LessThanOrEqual/2
  LessThanOrEqual/1 -> Switch/2
  Constant/1 -> Switch/3
  Constant1/1 -> Switch/1
  Switch/1 -> CTRL_wheelSlip_bool/1

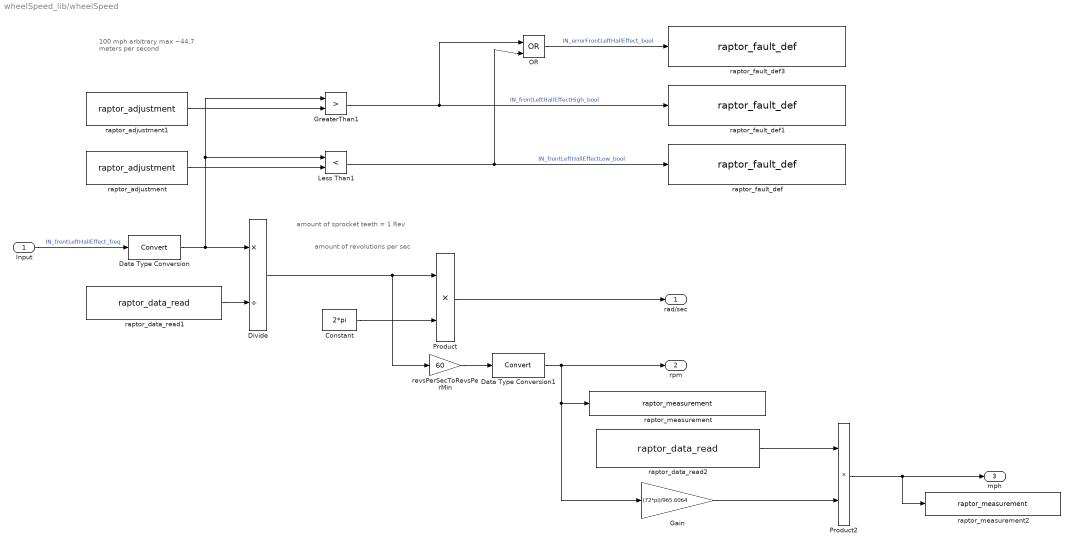
== system wheelSpeed_lib/wheelSpeed ==
  note: amount of revolutions per sec
  note: amount of sprocket teeth = 1 Rev
  note: 100 mph arbitrary max
      | ~44.7 meters per second
  Input : Inport
  Constant : Constant  Value=2*pi
  Data Type Conversion : DataTypeConversion  SaturateOnIntegerOverflow=off  RndMeth=Floor
  Data Type Conversion1 : DataTypeConversion  SaturateOnIntegerOverflow=off  RndMeth=Floor
  Divide : Product  Inputs=*/
  Gain : Gain  Gain=(72*pi)/965.6064
  GreaterThan1 : RelationalOperator  Operator=>  OutDataTypeStr=boolean  RndMeth=Simplest  InputSameDT=off
  Less Than1 : RelationalOperator  Operator=<  OutDataTypeStr=boolean  RndMeth=Simplest  InputSameDT=off
  OR : Logic  Operator=OR  IconShape=distinctive  AllPortsSameDT=off  OutDataTypeStr=boolean
  Product : Product
  Product2 : Product
  raptor_adjustment : Raptor_lib/Data Storage/raptor_adjustment  paramName=['IN_hallEffectLow' pos '_hz']  nameSource=Parameter  initValue=0  dataType=single  storage=Calibration  calDispType=Number  calEnum={'False', 'True'}  calGain=1.0  calOffset=0.0  calMax=inf  calMin=-inf  calFormat='-1'  calUnit=''  calHelp=''  calAccess=1  calFunction=raptor_xcp_function(gcb)  calDispHeaders=off  calColHeaders={'Col1' 'Col2' 'Col3'}  calRowHeaders={'Row1' 'Row2' 'Row3'}
      settings: SourceProductName=Raptor
  raptor_adjustment1 : Raptor_lib/Data Storage/raptor_adjustment  paramName=['IN_hallEffectHigh' pos '_hz']  nameSource=Parameter  initValue=1680  dataType=single  storage=Calibration  calDispType=Number  calEnum={'False', 'True'}  calGain=1.0  calOffset=0.0  calMax=inf  calMin=-inf  calFormat='-1'  calUnit=''  calHelp=''  calAccess=1  calFunction=raptor_xcp_function(gcb)  calDispHeaders=off  calColHeaders={'Col1' 'Col2' 'Col3'}  calRowHeaders={'Row1' 'Row2' 'Row3'}
      settings: SourceProductName=Raptor
  raptor_data_read1 : Raptor_lib/Data Storage/raptor_data_read  dataName='DATA_wheelTooth_ct'  dataShape=Scalar  idxSource=Input  idxRow=1  idxCol=1
      settings: SourceProductName=Raptor
  raptor_data_read2 : Raptor_lib/Data Storage/raptor_data_read  dataName='DATA_unloadedWheelRadius_m'  dataShape=Scalar  idxSource=Input  idxRow=1  idxCol=1
      settings: SourceProductName=Raptor
  raptor_fault_def : Raptor_lib/Faults/raptor_fault_def  faultName=['IN_hallEffectVLow' pos '_bool']  persist=off  sticky=off  emisRelated=off  singleTrip=off  clearMethod=Standard  xLimit=25  yLimit=50  calEnable=on  addDisable=off  calAccess=1  calFunction='System | FaultManager'
      settings: SourceProductName=Raptor
  raptor_fault_def1 : Raptor_lib/Faults/raptor_fault_def  faultName=['IN_hallEffectVHigh' pos '_bool']  persist=off  sticky=off  emisRelated=off  singleTrip=off  clearMethod=Standard  xLimit=25  yLimit=50  calEnable=on  addDisable=off  calAccess=1  calFunction='System | FaultManager'
      settings: SourceProductName=Raptor
  raptor_fault_def3 : Raptor_lib/Faults/raptor_fault_def  faultName=['IN_hallEffectError' pos '_bool']  persist=off  sticky=off  emisRelated=off  singleTrip=off  clearMethod=Standard  xLimit=25  yLimit=50  calEnable=on  addDisable=off  calAccess=1  calFunction='System | FaultManager'
      settings: SourceProductName=Raptor
  raptor_measurement : Raptor_lib/Data Storage/raptor_measurement  paramName=['IN_wheelSpeed' pos '_rpm']  nameSource=Parameter  calDispType=Number  calEnum={'False', 'True'}  calGain=1.0  calOffset=0.0  calMax=inf  calMin=-inf  calFormat='-1'  calUnit=''  calHelp=''  calAccess=1  calFunction=raptor_xcp_function(gcb)  calVisible=on
      settings: SourceProductName=Raptor
  raptor_measurement2 : Raptor_lib/Data Storage/raptor_measurement  paramName=['IN_wheelSpeed' pos '_mph']  nameSource=Parameter  calDispType=Number  calEnum={'False', 'True'}  calGain=1.0  calOffset=0.0  calMax=inf  calMin=-inf  calFormat='-1'  calUnit=''  calHelp=''  calAccess=1  calFunction=raptor_xcp_function(gcb)  calVisible=on
      settings: SourceProductName=Raptor
  revsPerSecToRevsPerMin : Gain  Gain=60
  rad/sec : Outport  OutDataTypeStr=double
  rpm : Outport  Port=2  OutDataTypeStr=double
  mph : Outport  Port=3
  wires:
  raptor_data_read1/1 -> Divide/2
  OR/1 -> raptor_fault_def3/1  "IN_errorFrontLeftHallEffect_bool"
  Constant/1 -> Product/2
  Input/1 -> Data Type Conversion/1  "IN_frontLeftHallEffect_freq"
  Less Than1/1 -> raptor_fault_def/1, OR/2  "IN_frontLeftHallEffectLow_bool"
  raptor_adjustment/1 -> Less Than1/2
  GreaterThan1/1 -> raptor_fault_def1/1, OR/1  "IN_frontLeftHallEffectHigh_bool"
  Product/1 -> rad/sec/1
  Divide/1 -> revsPerSecToRevsPerMin/1, Product/1
  revsPerSecToRevsPerMin/1 -> Data Type Conversion1/1
  raptor_adjustment1/1 -> GreaterThan1/2
  Data Type Conversion/1 -> Less Than1/1, GreaterThan1/1, Divide/1
  Product2/1 -> mph/1, raptor_measurement2/1
  Data Type Conversion1/1 -> rpm/1, Gain/1, raptor_measurement/1
  Gain/1 -> Product2/2
  raptor_data_read2/1 -> Product2/1
